simulink model "step_encoder_recording"  (R2018a)
settings: Solver=FixedStepDiscrete  StartTime=0.0  StopTime=10.0  RelTol=1e-3
PreLoadFcn:
  | waijung.modelPreload; % Required for working with Waijung Blockset. Do not remove.
undefined symbols (not defined in the file or in its folder): HSEOSC, Link, LQFP144, ST, STM32F446ZE
libraries: simulink x14, stm32f4_io_lib x7, commsynccomp2 x2, stm32f4_device_config_lib x1, dspbuff3 x1, stm32f4_tim_lib x1
(part 1 of 4)
CloseFcn:
  | waijung.modelClose; % Required for working with Waijung Blockset. Do not remove.
settings Model: Creator=Krisada  LastModifiedBy=izhak
settings DataIOCC: LimitDataPoints=on  SaveFormat=Array  SignalLoggingSaveFormat=ModelDataLogs
settings OptimizationCC: ExpressionDepthLimit=2147483647  LifeSpan=1
settings DebuggingCC: UnderspecifiedInitializationDetection=Classic  MergeDetectMultiDrivingBlocksExec=none  SolverPrmCheckMsg=warning  FcnCallInpInsideContextMsg=warning  StateNameClashWarn=warning  SFUnexpectedBacktrackingDiag=warning  SFNoUnconditionalDefaultTransitionDiag=warning  SFExecutionAtInitializationDiag=none
settings HardwareCC: ProdBitPerPointer=32  ProdBitPerSizeT=32  ProdBitPerPtrDiffT=32  ProdLargestAtomicFloat=None  ProdIntDivRoundTo=Undefined  ProdWordSize=32  ProdHWDeviceType=ARM Compatible->Cortex - M4  TargetEndianess=LittleEndian  TargetHWDeviceType=ARM Compatible->Cortex - M4
settings ModelReferenceCC: PropagateSignalLabelsOutOfModel=off
settings SFSimCC: MATLABDynamicMemAlloc=off
settings RTWCC: SystemTargetFile=stm32f4.tlc  GenerateMakefile=off  TemplateMakefile=ert_default_tmf  Description=STM32F4 Target
settings CodeAppCC: IgnoreCustomStorageClasses=off  CustomSymbolStrType=$N$R$M  StateflowObjectComments=on  InternalIdentifier=Classic
settings STFCustomTargetCC: ModelReferenceCompliant=off  CombineOutputUpdateFcns=on  ERTCustomFileBanners=on  SupportContinuousTime=off  SupportNonInlinedSFcns=off  RemoveResetFunc=on  MATLABClassNameForMDSCustomization=Simulink.SoftwareTarget.ERTCustomization  GRTInterface=off  SystemTargetFile=stm32f4.tlc
settings ERTTargetCC: MultiwordLength=2048  ModelReferenceCompliant=off  ParMdlRefBuildCompliant=off  CompOptLevelCompliant=off  ConcurrentExecutionCompliant=off  ModelStepFunctionPrototypeControlCompliant=off  CPPClassGenCompliant=off  UseToolchainInfoCompliant=off  ExtModeMexFile=noextcomm  ERTSrcFileBannerTemplate=stm32f4_code_template.cgt  ERTHdrFileBannerTemplate=stm32f4_code_template.cgt  ERTDataSrcFileTemplate=stm32f4_code_template.cgt  ERTDataHdrFileTemplate=stm32f4_code_template.cgt  ERTCustomFileTemplate=stm32f4_file_process.tlc  ConvertIfToSwitch=off  SuppressUnreachableDefaultCases=off
settings ConfigComp: CovMetricSettings=dw  CovHtmlReporting=on  CovSaveCumulativeToWorkspaceVar=on  CovSaveSingleToWorkspaceVar=on  CovExternalEMLEnable=off

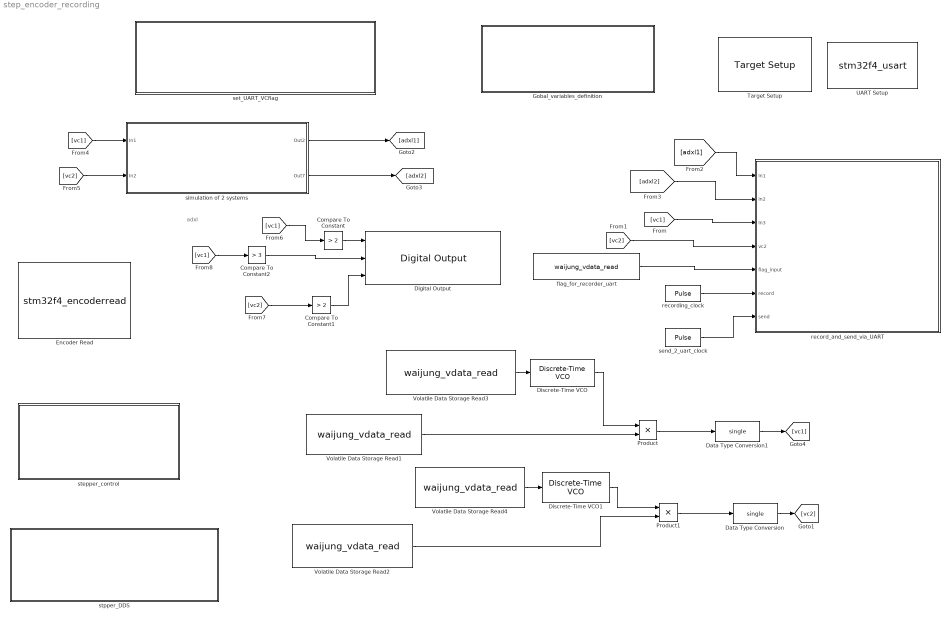
== system step_encoder_recording ==
  note: adxl
  Compare To Constant : simulink/Logic and Bit Operations/Compare To Constant  relop=>  const=2  OutDataTypeStr=boolean
  Compare To Constant1 : simulink/Logic and Bit Operations/Compare To Constant  relop=>  const=2  OutDataTypeStr=boolean
  Compare To Constant2 : simulink/Logic and Bit Operations/Compare To Constant  relop=>  const=3  OutDataTypeStr=boolean
  Data Type Conversion : DataTypeConversion  OutDataTypeStr=single
  Data Type Conversion1 : DataTypeConversion  OutDataTypeStr=single
  Digital Output : stm32f4_io_lib/Digital Output  use_bitband=on  port=B  speed=100  porttype=Push Pull  porttypestr=PP  use_pin0=on  use_pin1=off  use_pin2=off  use_pin3=off  use_pin4=off  use_pin5=off  use_pin6=off  use_pin7=on  use_pin8=off  use_pin9=off  use_pin10=off  use_pin11=off  use_pin12=off  use_pin13=off  use_pin14=on  use_pin15=off  pinstr=GPIO_Pin_0 | GPIO_Pin_7 | GPIO_Pin_14  usedpinarray="[1  0  0  0  0  0  0  1  0  0  0  0  0  0  1  0]"  bitbandingstr=|  sampletime=-1  sampletimestr=-1  blockid=DigitalOutput  enablecustomportlabel=off  globalinit=off  cinputportlabel=In1, In2  coutputportlabel=0
      | #define DigitalOutput_B0 Peripheral_BB(GPIOB->ODR, 0)  /* Output pin */
      | #define DigitalOutput_B7 Peripheral_BB(GPIOB->ODR, 7)  /* Output pin */
      | #define DigitalOutput_B14 Peripheral_BB(GPIOB->ODR, 14)  /* Output pin */
      settings: SourceProductName=Waijung Blockset
  Discrete-Time VCO : commsynccomp2/Discrete-Time VCO  Ac=1  Fc=0  Kc=1  Ph=0  ts=1e-3
      settings: SourceProductName=Communications System Toolbox  SourceProductBaseCode=CM
  Discrete-Time VCO1 : commsynccomp2/Discrete-Time VCO  Ac=1  Fc=0  Kc=1  Ph=0  ts=1e-3
      settings: SourceProductName=Communications System Toolbox  SourceProductBaseCode=CM
  Encoder Read : S-Function  FunctionName=stm32f4_encoderread  Parameters=sampletime,sampletimestr,blockid,timer,apb,portstr,pinstr,pinmat,chmat,filterstr,filter,factor,rstcnt,ppr  SFunctionDeploymentMode=off  EnableBusSupport=off  mask(stm32f4_encoderread){timer=1, ch1=E9, ch2=E11, ppr=500, rstcnt=off, filterstr=No filter; sampling is done at fDTS, sampletime=-1, sampletimestr=-1, blockid=EncoderRead, absresetinput=off, portpinstr=,, portstr=[], pinstr=[], pinmat=zeros(0,1), chmat=[], apb=0, filter=0, factor=4}
      mask prompts: ch1 "Channel A Input Pin"; ch2 "Channel B Input Pin"; ppr "PPR (Number of pulses generated per revolution)"; rstcnt "Reset counter after every counter read"; filterstr "Built-in Input Capture Filter"; sampletime "Sample time (sec)"; sampletimestr "Compiled sample time (sec) in string"; absresetinput "Enable absolute position reset input signal"; portpinstr "Port pin string"; portstr "Port string"; pinstr "Pin string"; pinmat "Pin matrix"; chmat "Channel order"; filter "Filter ID"
      mask help:
      | The output Direction (uint32) is the direction of rotation either 0 or 1.
      |
      | The output Position (count) (uint32) is the count of number of edges of the encoder output signals from either channel A and B. The decoder is set to count at every rising and falling edge of both channel A and B (4x) or (x2) for one channel. For example, if an encoder has 180 pulses per revolution (PPS) and two channels are selected, the maximum count is 720 per revolution (4x180 = 720), i.e. from 0 to 719.
      mask init:
      | stm32f4_encoderread_callback('init');
      mask Help: web(fullfile(waijungdocroot,'stm32f4_encoderread.htm'),'-browser')
      mask TypeOptions timer: 1 | 2 | 3 | 4 | 5 | 8
      mask Callback timer: stm32f4_encoderread_callback('timer');
      mask TypeOptions ch1: Not available - Do not use | E9 | A8
      mask Callback ch1: stm32f4_encoderread_callback('chA');
      mask TypeOptions ch2: Not available - Do not use | E11 | A9
      mask Callback ch2: stm32f4_encoderread_callback('chB');
      mask Callback ppr: stm32f4_encoderread_callback('ppr');
      mask Callback rstcnt: stm32f4_encoderread_callback('rstcnt');
      mask TypeOptions filterstr: No filter; sampling is done at fDTS | fSAMPLING=fCK_INT; N=2 | fSAMPLING=fCK_INT; N=4 | fSAMPLING=fCK_INT; N=8 | fSAMPLING=fDTS/2; N=6 | fSAMPLING=fDTS/2; N=8 | fSAMPLING=fDTS/4; N=6 | fSAMPLING=fDTS/4; N=8 | fSAMPLING=fDTS/8; N=6 | fSAMPLING=fDTS/8; N=8 | fSAMPLING=fDTS/16; N=5 | fSAMPLING=fDTS/16; N=6 | fSAMPLING=fDTS/16; N=8 | fSAMPLING=fDTS/32; N=5 | fSAMPLING=fDTS/32; N=6 | fSAMPLING=fDTS/32; N=8
      mask Callback filterstr: stm32f4_encoderread_callback('filterstr');
      mask Callback sampletimestr: stm32f4_encoderread_callback('sampletimestr');
      mask Callback blockid: stm32f4_encoderread_callback('blockid');
      mask Display: text(0.05, 0.5, 'Timer: 1\nInput pins [CH_A, CH_B]: [-,-]\nRST Counter: No\nTs (sec): -1','ver','middle','hor','left');port_label('output', 1, 'Direction');port_label('output', 2, 'Position (count)')
  Gobal_variables_definition : Subsystem
  Product : Product
  Product1 : Product
  Target Setup : stm32f4_device_config_lib/Target Setup  Priority=1  compiler=GNU ARM  previous_compiler=GNU ARM  mcu=STM32F446ZE (LQFP144)  mcustr=STM32F446ZE  clockconfig=HSEOSC-8MHz  system_stm32f4xx_c_path=C:\MATLAB\waijung17_03a\targets\stm32f4_target\stm32f4\utils\system_stm32f4xx_default\STM32F446xx\hseosc8mhz  showmemoryconfiguration=off  stacksize=0x400  heapsize=0x200  enableautocompiledownload=on  fullchiperase=off  programmerinterface=ST-Link  editctrlstr=on  compilercontrolstr=$(patsubst %, -I%, .) -mcpu=cortex-m4 -mthumb -mthumb-interwork -mfloat-abi=hard -mfpu=fpv4-sp-d16 -ffast-math -Wall -Wextra -Ofast  assemblercontrolstr=$(patsubst %, -I%, .) -mcpu=cortex-m4 -mthumb -mthumb-interwork -mfloat-abi=hard -mfpu=fpv4-sp-d16 -ffast-math -Wall -Wextra -Ofast -Wa,-amhls=$(<:.s=.lst) -D__STACK_SIZE=$(STACK_SIZE) -D__HEAP_SIZE=$(HEAP_SIZE)  linkercontrolstr=-T$(LD_SCRIPT) -g -Wl,-Map=$(MAP),--cref,--no-warn-mismatch -mcpu=cortex-m4 -mthumb -mthumb-interwork -mfloat-abi=hard -mfpu=fpv4-sp-d16 -specs=nosys.specs  runafterdownload=on  execprofile=None  profileruart=1  profilerbaud=115200  profilertxpin=D8  profilerinitstr=0.001,180000000,180000,115200,0  manualsetsampletime=on  sampletime=0.001  blockid=TargetSetup  systickreloadvalue=180000  hseval=8000000  lastprofileruart=1  hclk=180000000  flashorigin=0x8000000  flashlength=512k  ramorigin=0x20000000  ramlength=128k  useextram=off
      settings: SourceProductName=Waijung Blockset
  UART Setup : S-Function  Priority=1  FunctionName=stm32f4_usart  Parameters=configuration,uartmodule,transfer,baudrate,inputtype,outputtype,confstr,binheaderarray,binterminatorarray,asciiheader,asciiterminator,bindatalength,packetmode,varname,sampletime,sampletimestr,blockid  SFunctionDeploymentMode=off  EnableBusSupport=off  mask(stm32f4_usart){configuration=Setup, uartmodule=3, baudrate=115200, databits=8, parity=No, stopbit=1, remaptxpin=D8, remaprxpin=D9, flowcontrol=None, remapctspin=Not used, remaprtspin=Not used, advanceoptions=off, rxbuffersize=512, txbuffersize=512, transfer=Blocking, packetmode=Ascii, binheader='7E 7E', binterminator='03 03', porttype_double=1, porttype_single=0, porttype_int8=1, porttype_uint8=0, porttype_int16=0, porttype_uint16=0, porttype_int32=0, porttype_uint32=0, asciiformat='%d,%f', rx_asciiterminator=CRLF (0x0D 0x0A - "\r\n"), tx_asciiterminator=CR (0x0D - "\r"), storagename=<empty>, varname=, inputtype=[0], outputtype=[0], binheaderarray=[0], binterminatorarray=[0], bindatalength=0, asciiheader='', asciiterminator=[0], sampletime=-1, sampletimestr=-1, blockid=UARTSetup, confstr=[ "dummy", "1", "D", "8", "1", "D", "9", "0", "*", "*", "0", "*", "*", "1", "4", "3", "1", "4", "1", "512", "512", "1", "3", "115200", "8", "No", "1", "None", "USART3"], lastmodule=3}
      mask prompts: uartmodule "UART Module"; baudrate "Baud rate (bps)"; databits "Data bits"; stopbit "Stop bit"; remaptxpin "Tx Pin"; remaprxpin "Rx Pin"; flowcontrol "Hardware flow control"; remapctspin "HW Flow control, CTS Pin"; remaprtspin "HW Flow control, RTS Pin"; advanceoptions "Advance options"; rxbuffersize "Rx buffer size (bytes)"; txbuffersize "Tx buffer size (bytes)"; packetmode "Packet mode"; binheader "Binary header (example: '7E 7E')"; binterminator "Binary terminator (example: '03 03')"; porttype_double "Number of data port, type DOUBLE"; porttype_single "Number of data port, type SINGLE"; porttype_int8 "Number of data port, type INT8"; porttype_uint8 "Number of data port, type UINT8"; porttype_int16 "Number of data port, type INT16"; porttype_uint16 "Number of data port, type UINT16"; porttype_int32 "Number of data port, type INT32"; porttype_uint32 "Number of data port, type UINT32"; asciiformat "Ascii format"; rx_asciiterminator "End of packet"; tx_asciiterminator "End of packet"; storagename "Buffer"; varname "Var name"; inputtype "Input data type"; outputtype "Output data type"; binheaderarray "Binary header"; binterminatorarray "Binary terminator"; bindatalength "Binary data length"; asciiheader "Ascii header (printf format)"; asciiterminator "Ascii terminator"; sampletime "Sample time (sec)"; sampletimestr "Compiled sample time (sec) in string"; confstr "Configuration string"; lastmodule "Last module selected"
      mask init:
      | stm32f4_usart_callback('init');
      mask Help: web(fullfile(waijungdocroot,'stm32f4_usart_setup.htm'), '-browser')
      mask TypeOptions configuration: Setup | Tx | Rx
      mask Callback configuration: stm32f4_usart_callback('configuration');
      mask TypeOptions uartmodule: 1 | 2 | 3 | 4 | 5 | 6
      mask Callback uartmodule: stm32f4_usart_callback('uartmodule');
      mask Callback baudrate: stm32f4_usart_callback('baudrate');
      mask TypeOptions databits: 8
      mask TypeOptions parity: No | Odd | Even
      mask TypeOptions stopbit: 0.5 | 1 | 1.5 | 2
      mask TypeOptions remaptxpin: Not used | B10 | C10 | D8
      mask TypeOptions remaprxpin: Not used | B11 | C11 | D9
      mask TypeOptions flowcontrol: None | RTS | CTS | RTS/CTS
      mask Callback flowcontrol: stm32f4_usart_callback('flowcontrol');
      mask TypeOptions remapctspin: Not used | B13 | D11
      mask TypeOptions remaprtspin: Not used | B14 | D12
      mask Callback advanceoptions: stm32f4_usart_callback('advanceoptions');
      mask TypeOptions rxbuffersize: 16 | 32 | 64 | 128 | 256 | 512 | 1024 | 2048
      mask TypeOptions txbuffersize: 16 | 32 | 64 | 128 | 256 | 512 | 1024 | 2048
      mask TypeOptions transfer: Blocking | Non-Blocking
      mask Callback transfer: stm32f4_usart_callback('transfer');
      mask TypeOptions packetmode: Ascii | Binary | String Buffer
      mask Callback packetmode: stm32f4_usart_callback('packetmode');
      mask Callback binheader: stm32f4_usart_callback('binheader');
      mask Callback binterminator: stm32f4_usart_callback('binterminator');
      mask Callback porttype_double: stm32f4_usart_callback('porttype');
      mask Callback porttype_single: stm32f4_usart_callback('porttype');
      mask Callback porttype_int8: stm32f4_usart_callback('porttype');
      mask Callback porttype_uint8: stm32f4_usart_callback('porttype');
      mask Callback porttype_int16: stm32f4_usart_callback('porttype');
      mask Callback porttype_uint16: stm32f4_usart_callback('porttype');
      mask Callback porttype_int32: stm32f4_usart_callback('porttype');
      mask Callback porttype_uint32: stm32f4_usart_callback('porttype');
      mask Callback asciiformat: stm32f4_usart_callback('asciiformat');
      mask TypeOptions rx_asciiterminator: CR (0x0D - "\r") | LF (0x0A - "\n") | CRLF (0x0D 0x0A - "\r\n")
      mask Callback rx_asciiterminator: stm32f4_usart_callback('rx_asciiterminator');
      mask TypeOptions tx_asciiterminator: CR (0x0D - "\r") | LF (0x0A - "\n") | CRLF (0x0D 0x0A - "\r\n") | None
      mask Callback tx_asciiterminator: stm32f4_usart_callback('tx_asciiterminator');
      mask TypeOptions storagename: <empty>
      mask Callback storagename: stm32f4_usart_callback('storagename');
      mask Callback varname: stm32f4_usart_callback('varname');
      mask Callback sampletime: stm32f4_usart_callback('sampletime');
      mask Callback sampletimestr: stm32f4_usart_callback('sampletimestr');
      mask Callback blockid: stm32f4_usart_callback('blockid');
      mask Display: text(0.5, 0.5, 'Module: USART3_Setup\nBaud (Bps): 115200\nDMA Buffer: 512/512\nTx/Rx Pin: D8/D9','ver','middle','hor','center');
  Volatile Data Storage Read1 : S-Function  FunctionName=waijung_vdata_read  Parameters=storagename,varname,sampletime,sampletimestr,blockid,storagetype,storagetypestr  SFunctionDeploymentMode=off  EnableBusSupport=off  mask(waijung_vdata_read){storagename=Ax, varname=Gobal_variables_definitionVolatileDataStorage2_Ax, sampletime=.001, sampletimestr=-1, blockid=VolatileDataStorageRead1, storagetype=double, storagetypestr=double}
      mask prompts: storagename "Storage Name"; varname "Variable name"; sampletime "Sample time (sec)"; sampletimestr "Compiled sample time (sec) in string"; storagetype "Data type"; storagetypestr "Data type string"
      mask help: This block implements read data from a buffer.
      mask init:
      | waijung_vdata_read_callback('init');
      mask Help: web(fullfile(waijungdocroot,'Volatile_Data_Storage_Read.htm'))
      mask TypeOptions storagename: Laser | Ax | flag | fx | fy | Ay
      mask Callback storagename: waijung_vdata_read_callback('storagename');
      mask Callback varname: waijung_vdata_read_callback('varname');
      mask Callback sampletime: waijung_vdata_read_callback('sampletime');
      mask Callback sampletimestr: waijung_vdata_read_callback('sampletimestr');
      mask Callback blockid: waijung_vdata_read_callback('blockid');
      mask Callback storagetype: waijung_vdata_read_callback('storagetype');
      mask Display: text(0.05, 0.5, 'Buffer: Ax','ver','middle','hor','left');port_label('output',1,'D1(double)')
  Volatile Data Storage Read2 : S-Function  FunctionName=waijung_vdata_read  Parameters=storagename,varname,sampletime,sampletimestr,blockid,storagetype,storagetypestr  SFunctionDeploymentMode=off  EnableBusSupport=off  mask(waijung_vdata_read){storagename=Ay, varname=Gobal_variables_definitionVolatileDataStorage6_Ay, sampletime=.001, sampletimestr=-1, blockid=VolatileDataStorageRead2, storagetype=double, storagetypestr=double}
      mask prompts: storagename "Storage Name"; varname "Variable name"; sampletime "Sample time (sec)"; sampletimestr "Compiled sample time (sec) in string"; storagetype "Data type"; storagetypestr "Data type string"
      mask help: This block implements read data from a buffer.
      mask init:
      | waijung_vdata_read_callback('init');
      mask Help: web(fullfile(waijungdocroot,'Volatile_Data_Storage_Read.htm'))
      mask TypeOptions storagename: Laser | Ax | flag | fx | fy | Ay
      mask Callback storagename: waijung_vdata_read_callback('storagename');
      mask Callback varname: waijung_vdata_read_callback('varname');
      mask Callback sampletime: waijung_vdata_read_callback('sampletime');
      mask Callback sampletimestr: waijung_vdata_read_callback('sampletimestr');
      mask Callback blockid: waijung_vdata_read_callback('blockid');
      mask Callback storagetype: waijung_vdata_read_callback('storagetype');
      mask Display: text(0.05, 0.5, 'Buffer: Ay','ver','middle','hor','left');port_label('output',1,'D1(double)')
  Volatile Data Storage Read3 : S-Function  FunctionName=waijung_vdata_read  Parameters=storagename,varname,sampletime,sampletimestr,blockid,storagetype,storagetypestr  SFunctionDeploymentMode=off  EnableBusSupport=off  mask(waijung_vdata_read){storagename=fx, varname=Gobal_variables_definitionVolatileDataStorage4_fx, sampletime=.001, sampletimestr=-1, blockid=VolatileDataStorageRead3, storagetype=double, storagetypestr=double}
      mask prompts: storagename "Storage Name"; varname "Variable name"; sampletime "Sample time (sec)"; sampletimestr "Compiled sample time (sec) in string"; storagetype "Data type"; storagetypestr "Data type string"
      mask help: This block implements read data from a buffer.
      mask init:
      | waijung_vdata_read_callback('init');
      mask Help: web(fullfile(waijungdocroot,'Volatile_Data_Storage_Read.htm'))
      mask TypeOptions storagename: Laser | Ax | flag | fx | fy | Ay
      mask Callback storagename: waijung_vdata_read_callback('storagename');
      mask Callback varname: waijung_vdata_read_callback('varname');
      mask Callback sampletime: waijung_vdata_read_callback('sampletime');
      mask Callback sampletimestr: waijung_vdata_read_callback('sampletimestr');
      mask Callback blockid: waijung_vdata_read_callback('blockid');
      mask Callback storagetype: waijung_vdata_read_callback('storagetype');
      mask Display: text(0.05, 0.5, 'Buffer: fx','ver','middle','hor','left');port_label('output',1,'D1(double)')
  Volatile Data Storage Read4 : S-Function  FunctionName=waijung_vdata_read  Parameters=storagename,varname,sampletime,sampletimestr,blockid,storagetype,storagetypestr  SFunctionDeploymentMode=off  EnableBusSupport=off  mask(waijung_vdata_read){storagename=fy, varname=Gobal_variables_definitionVolatileDataStorage5_fy, sampletime=.001, sampletimestr=-1, blockid=VolatileDataStorageRead4, storagetype=double, storagetypestr=double}
      mask prompts: storagename "Storage Name"; varname "Variable name"; sampletime "Sample time (sec)"; sampletimestr "Compiled sample time (sec) in string"; storagetype "Data type"; storagetypestr "Data type string"
      mask help: This block implements read data from a buffer.
      mask init:
      | waijung_vdata_read_callback('init');
      mask Help: web(fullfile(waijungdocroot,'Volatile_Data_Storage_Read.htm'))
      mask TypeOptions storagename: Laser | Ax | flag | fx | fy | Ay
      mask Callback storagename: waijung_vdata_read_callback('storagename');
      mask Callback varname: waijung_vdata_read_callback('varname');
      mask Callback sampletime: waijung_vdata_read_callback('sampletime');
      mask Callback sampletimestr: waijung_vdata_read_callback('sampletimestr');
      mask Callback blockid: waijung_vdata_read_callback('blockid');
      mask Callback storagetype: waijung_vdata_read_callback('storagetype');
      mask Display: text(0.05, 0.5, 'Buffer: fy','ver','middle','hor','left');port_label('output',1,'D1(double)')
  flag_for_recorder_uart : S-Function  FunctionName=waijung_vdata_read  Parameters=storagename,varname,sampletime,sampletimestr,blockid,storagetype,storagetypestr  SFunctionDeploymentMode=off  EnableBusSupport=off  mask(waijung_vdata_read){storagename=flag, varname=Gobal_variables_definitionVolatileDataStorage3_flag, sampletime=1e-3, sampletimestr=-1, blockid=flag_for_recorder_uart, storagetype=uint8, storagetypestr=uint8_t}
      mask prompts: storagename "Storage Name"; varname "Variable name"; sampletime "Sample time (sec)"; sampletimestr "Compiled sample time (sec) in string"; storagetype "Data type"; storagetypestr "Data type string"
      mask help: This block implements read data from a buffer.
      mask init:
      | waijung_vdata_read_callback('init');
      mask Help: web(fullfile(waijungdocroot,'Volatile_Data_Storage_Read.htm'))
      mask TypeOptions storagename: Laser | Ax | flag | fx | fy | Ay
      mask Callback storagename: waijung_vdata_read_callback('storagename');
      mask Callback varname: waijung_vdata_read_callback('varname');
      mask Callback sampletime: waijung_vdata_read_callback('sampletime');
      mask Callback sampletimestr: waijung_vdata_read_callback('sampletimestr');
      mask Callback blockid: waijung_vdata_read_callback('blockid');
      mask Callback storagetype: waijung_vdata_read_callback('storagetype');
      mask Display: text(0.05, 0.5, 'Buffer: flag','ver','middle','hor','left');port_label('output',1,'D1(uint8)')
  record_and_send_via_UART : Subsystem
  recording_clock : DiscretePulseGenerator  SampleTime=1e-3
  send_2_uart_clock : DiscretePulseGenerator  SampleTime=1e-3
  set_UART_VCflag : Subsystem
  simulation of 2 systems : Subsystem
  stepper_control : Subsystem
  stpper_DDS : Subsystem
  wires:
  flag_for_recorder_uart/1 -> record_and_send_via_UART/5(flag_input)
  recording_clock/1 -> record_and_send_via_UART/6(record)
  send_2_uart_clock/1 -> record_and_send_via_UART/7(send)
  [vc1] -> record_and_send_via_UART/3(In3)
  [vc2] -> record_and_send_via_UART/4(vc2)
  [adxl1] -> record_and_send_via_UART/1(In1)
  [adxl2] -> record_and_send_via_UART/2(In2)
  Data Type Conversion/1 -> [vc2]
  Data Type Conversion1/1 -> [vc1]
  Product/1 -> Data Type Conversion1/1
  Discrete-Time VCO/1 -> Product/1
  Volatile Data Storage Read1/1 -> Product/2
  simulation of 2 systems/1(Out2) -> [adxl1]
  simulation of 2 systems/2(Out7) -> [adxl2]
  Volatile Data Storage Read3/1 -> Discrete-Time VCO/1
  Volatile Data Storage Read4/1 -> Discrete-Time VCO1/1
  Volatile Data Storage Read2/1 -> Product1/2
  Discrete-Time VCO1/1 -> Product1/1
  Product1/1 -> Data Type Conversion/1
  [vc1] -> simulation of 2 systems/1(In1)
  [vc2] -> simulation of 2 systems/2(In2)
  [vc1] -> Compare To Constant/1
  Compare To Constant/1 -> Digital Output/1
  [vc2] -> Compare To Constant1/1
  Compare To Constant1/1 -> Digital Output/3
  [vc1] -> Compare To Constant2/1
  Compare To Constant2/1 -> Digital Output/2
